simulink model "UEESP2015a"  (R2015a)
settings: Solver=ode45  SolverMode=SingleTasking  StartTime=0.0  StopTime=10.0  RelTol=1e-3
values from neighbouring files (symbols this model uses):
  A = [0 1 0 0;-c_ds/J_1-c_ds/J_2 -b_1/J_1 -b_1/J_1+b_2/J_2 -i_rori/J_2;c_ds/J_2 0 -b_2/J_2 i_rori/J_2;0 0 0 -1/tau]    [UE_08_Reglerentwurf_EPS.m]
  B_sim = [E B]    [UE_08_Reglerentwurf_EPS.m]
  C = [c_ds 0 0 0;0 0 i_rori 0]    [UE_08_Reglerentwurf_EPS.m]
  C_sim = eye(4)    [UE_08_Reglerentwurf_EPS.m]
  D_sim = [0 0 0;0 0 0;0 0 0;0 0 0]    [UE_08_Reglerentwurf_EPS.m]
  K_PZ = [0 0 0 0]    [UE_08_Reglerentwurf_EPS.m]
  x0 = [2*pi/180 0 0 0]'    [UE_08_Reglerentwurf_EPS.m]
settings Model: CovMetricSettings=dwe  CovHtmlReporting=off  covSaveCumulativeToWorkspaceVar=off  CovSaveSingleToWorkspaceVar=off  CovExternalEMLEnable=on  Creator=Jason  LastModifiedBy=Jason
settings DataIOCC: LimitDataPoints=off  SaveFormat=Dataset
settings DebuggingCC: SFUnexpectedBacktrackingDiag=error  SFNoUnconditionalDefaultTransitionDiag=error
settings HardwareCC: ProdBitPerPointer=64  ProdLargestAtomicFloat=Float  ProdIntDivRoundTo=Zero  ProdEndianess=LittleEndian  ProdHWDeviceType=Specified
settings ModelReferenceCC: PropagateSignalLabelsOutOfModel=on
settings GRTTargetCC: TargetLangStandard=C99 (ISO)  GeneratePreprocessorConditionals=Use local settings

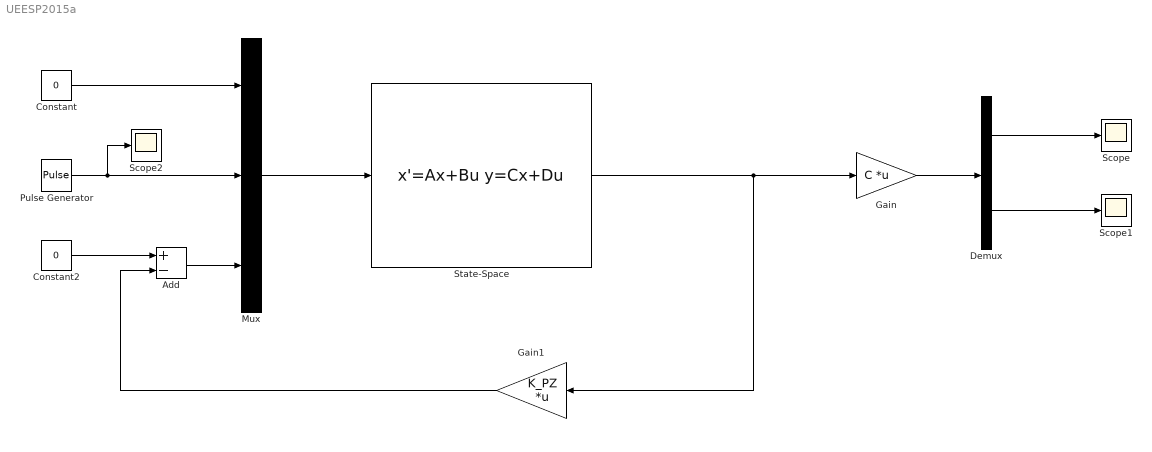
== system UEESP2015a ==
  Add : Sum  Inputs=+-
  Constant : Constant  Value=0
  Constant2 : Constant  Value=0
  Demux : Demux  Outputs=2
  Gain : Gain  Gain=C  Multiplication=Matrix(K*u)
  Gain1 : Gain  Gain=K_PZ  Multiplication=Matrix(K*u)
  Mux : Mux  Inputs=3
  Pulse Generator : DiscretePulseGenerator  PulseType=Time based  Period=10  PulseWidth=5
  Scope : Scope
      settings: TimeRange=auto  MaxDataPoints=5000  SaveToWorkspace=off  SaveName=ScopeData  YMin=-3.74865  YMax=3.90718  SampleTime=-1
  Scope1 : Scope
      settings: TimeRange=auto  MaxDataPoints=5000  SaveToWorkspace=off  YMin=-10  YMax=10  SampleTime=-1
  Scope2 : Scope
      settings: TimeRange=auto  MaxDataPoints=5000  SaveToWorkspace=off  SaveName=ScopeData2  YMin=-0.125  YMax=1.125  SampleTime=-1
  State-Space : StateSpace  A=A  B=B_sim  C=C_sim  D=D_sim  X0=x0
  wires:
  Constant/1 -> Mux/1
  Mux/1 -> State-Space/1
  Pulse Generator/1 -> Scope2/1, Mux/2
  Constant2/1 -> Add/1
  State-Space/1 -> Gain1/1, Gain/1
  Demux/2 -> Scope1/1
  Gain1/1 -> Add/2
  Demux/1 -> Scope/1
  Gain/1 -> Demux/1
  Add/1 -> Mux/3
